simulink model "semitrailer_state_space_model"  (R2013b)
settings: Solver=ode45  StartTime=0.0  StopTime=100  RelTol=1e-3
values from neighbouring files (symbols this model uses):
  CC = ft2/max(A2)    [semi_trailer_force.m]
  dy = 0.007    [semitrailer_sis.m]
  Lt11 = 4.8    [semitrailer_sis.m]
  Lt12 = 1.2    [semitrailer_sis.m]
  Lt13 = 3.6    [semitrailer_sis.m]
  Lt16 = 4.134    [semitrailer_sis.m]
  Lt21 = 4    [semitrailer_sis.m]
  Lt22 = 0.685    [semitrailer_sis.m]
  Lt23 = 0.7    [semitrailer_sis.m]
  Lt26 = 6.973    [semitrailer_sis.m]
  Vt = 60/3.6    (= 16.6666666667)    [semitrailer_sis.m]
  wt = Vt/dy    (= 2380.95238095)    [semitrailer_sis.m]
undefined symbols (not defined in the file or in its folder): A, B, D, get
libraries: dspxfrm3 x1, dspsnks4 x1, dspsigops x1
settings Model: Creator=oguzhan  LastModifiedBy=oguzhan

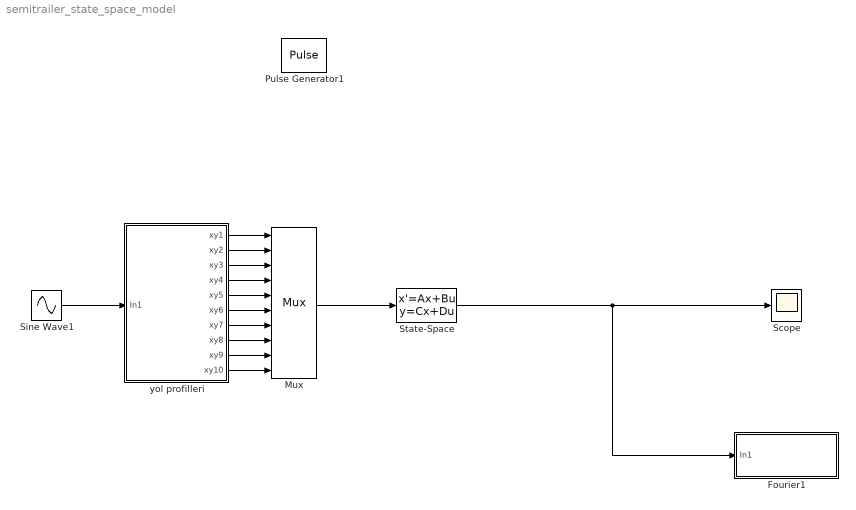
== system semitrailer_state_space_model ==
  Fourier1 : Subsystem
  Mux : Mux  Inputs=10
  Pulse Generator1 : DiscretePulseGenerator  PulseType=Time based  Amplitude=-0.01  Period=0.5  PulseWidth=0.025
  Scope : Scope
      settings: ShowLegends=on  MaxDataPoints=500000
  Sine Wave1 : Sin  Amplitude=dy  Frequency=wt*2*pi  SampleTime=0
  State-Space : StateSpace  A=A  B=B  C=CC  D=D  X0=0
  yol profilleri : Subsystem
  wires:
  yol profilleri/1(xy1) -> Mux/1
  yol profilleri/2(xy2) -> Mux/2
  yol profilleri/3(xy3) -> Mux/3
  yol profilleri/4(xy4) -> Mux/4
  yol profilleri/5(xy5) -> Mux/5
  yol profilleri/6(xy6) -> Mux/6
  yol profilleri/7(xy7) -> Mux/7
  yol profilleri/8(xy8) -> Mux/8
  yol profilleri/9(xy9) -> Mux/9
  yol profilleri/10(xy10) -> Mux/10
  Mux/1 -> State-Space/1
  State-Space/1 -> Fourier1/1(In1), Scope/1
  Sine Wave1/1 -> yol profilleri/1(In1)

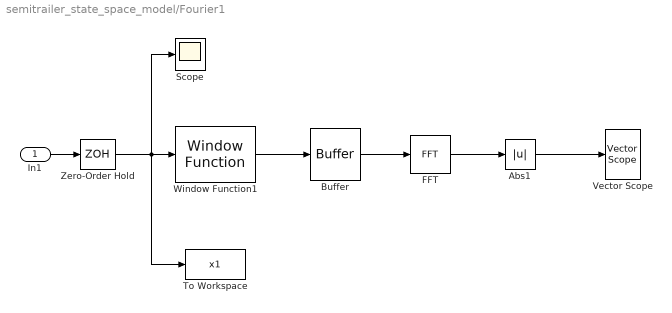
== system semitrailer_state_space_model/Fourier1 ==
  In1 : Inport
  Abs1 : Abs
  Buffer : Buffer  N=2^10  TreatMby1Signals=One channel
  FFT : dspxfrm3/FFT  CompMethod=Table lookup  TableOpt=NEW  TableOptActive=Speed  BitRevOrder=off  InheritFFTLength=on  FFTLength=2048  RowConvenienceOn=on  FFTImplementation=FFTW  SkipNorm=on  firstCoeffDataTypeStr=Inherit: Same word length as input  firstCoeffLastDataTypeStr=Inherit: Same word length as input  outputMin=[]  outputMax=[]  roundingMode=Floor  overflowMode=off
  Scope : Scope
      settings: ShowLegends=on  MaxDataPoints=500000
  To Workspace : ToWorkspace  VariableName=x1  SampleTime=-1
  Vector Scope : dspsnks4/Vector Scope  ScopeProperties=on  Domain=Frequency  HorizSpan=1  DisplayProperties=off  AxisGrid=on  Memory=off  FrameNumber=on  AxisLegend=off  AxisZoom=off  OpenScopeAtSimStart=on  OpenScopeImmediately=off  FigPos=get(0,'defaultfigureposition')  AxisProperties=off  XUnits=Hertz  XRange=[0...Fs/2]  InheritXIncr=on  XIncr=1  XLabel=Time  XLimit=Auto  XMin=0  XMax=300  XStart=0  YUnits=dB  YLabel=Amplitude  LineProperties=off  XAxisParamsVer=6.9
      settings: YMin=-100  YMax=-50
  Window Function1 : dspsigops/Window Function  winmode=Apply window to input  wintype=Hamming  sampmode=Continuous  samptime=1  N=64  Rs=50  beta=10  winsamp=Symmetric  UserWindow=hamming  OptParams=off  UserParams={'symmetric'}  RowConvenienceOn=on  dataType=double  isSigned=on  wordLen=16  udDataType=sfix(16)  fracBitsMode=Best precision  numFracBits=15  roundingMode=Floor  overflowMode=off  numSidelobes=4  sidelobeLevel=-30
  Zero-Order Hold : ZeroOrderHold  SampleTime=1/100
  wires:
  Buffer/1 -> FFT/1
  FFT/1 -> Abs1/1
  In1/1 -> Zero-Order Hold/1
  Zero-Order Hold/1 -> Scope/1, To Workspace/1, Window Function1/1
  Window Function1/1 -> Buffer/1
  Abs1/1 -> Vector Scope/1

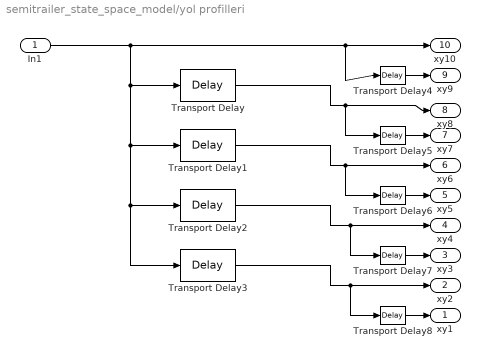
== system semitrailer_state_space_model/yol profilleri ==
  In1 : Inport
  Transport Delay : TransportDelay  DelayTime=(Lt12+Lt13)/Vt
  Transport Delay1 : TransportDelay  DelayTime=(Lt12+Lt11)/Vt
  Transport Delay2 : TransportDelay  DelayTime=(Lt12+Lt16+Lt26+Lt21-Lt22)/Vt
  Transport Delay3 : TransportDelay  DelayTime=(Lt12+Lt16+Lt26+Lt21+Lt23)/Vt
  Transport Delay{4..8} (5 alike) : TransportDelay  DelayTime=0.001
  xy1 : Outport
  xy2 : Outport  Port=2
  xy3 : Outport  Port=3
  xy4 : Outport  Port=4
  xy5 : Outport  Port=5
  xy6 : Outport  Port=6
  xy7 : Outport  Port=7
  xy8 : Outport  Port=8
  xy9 : Outport  Port=9
  xy10 : Outport  Port=10
  wires:
  In1/1 -> Transport Delay2/1, Transport Delay3/1, Transport Delay1/1, Transport Delay/1, xy10/1, Transport Delay4/1
  Transport Delay/1 -> xy8/1, Transport Delay5/1
  Transport Delay1/1 -> xy6/1, Transport Delay6/1
  Transport Delay2/1 -> xy4/1, Transport Delay7/1
  Transport Delay3/1 -> xy2/1, Transport Delay8/1
  Transport Delay4/1 -> xy9/1
  Transport Delay5/1 -> xy7/1
  Transport Delay6/1 -> xy5/1
  Transport Delay7/1 -> xy3/1
  Transport Delay8/1 -> xy1/1
